simulink model "Lapsim2"  (R2020a)
settings: Solver=VariableStepAuto  StartTime=0.0  StopTime=10  RelTol=1e-3
values from neighbouring files (symbols this model uses):
  Ap = A + B*[k1 k2 k3]    [Lapunow.m]
  B = [0 ; 0 ; 50]    [Lapunow.m]
settings Model: Creator=SARIS  LastModifiedBy=grzyb

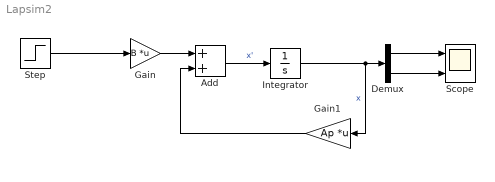
== system Lapsim2 ==
  Add : Sum
  Demux : Demux  Outputs=2
  Gain : Gain  Gain=B  Multiplication=Matrix(K*u)
  Gain1 : Gain  Gain=Ap  Multiplication=Matrix(K*u)
  Integrator : Integrator
  Scope : Scope  NumInputPorts=2
  Step : Step  SampleTime=0
  wires:
  Step/1 -> Gain/1
  Gain/1 -> Add/1
  Add/1 -> Integrator/1  "x'"
  Gain1/1 -> Add/2
  Integrator/1 -> Demux/1, Gain1/1  "x"
  Demux/1 -> Scope/1
  Demux/2 -> Scope/2
